simulink model "sim_MPC_Heli"  (R2020a)
settings: Solver=ode4  StartTime=0.0  StopTime=inf  FixedStep=0.01  RelTol=1e-3
InitFcn:
  | run('initialize_system.m')
values from neighbouring files (symbols this model uses):
  Ac = [d_f1_dth,d_f1_dyw,d_f1_dw_th,d_f1_dw_yw ... (first row only)    [linearize_heli.m]
  Ad = ds.a    [initialize_system.m]
  Bc = [d_f1_Vmp,d_f1_Vmy ... (first row only)    [linearize_heli.m]
  Bd = ds.b    [initialize_system.m]
  Cc = [1,0,0,0;0,1,0,0]    [linearize_heli.m]
  Cd = ds.c    [initialize_system.m]
  th_op = -10*pi/180    (= -0.174532925199)    [initialize_system.m]
  Vmp_op = (Kyy*m_heli*g*cos(th_op)*l_cm) / (Kyy*Kpp - Kyp*Kpy)    [initialize_system.m]
  Vmy_op = (Kyp*Vmp_op) / (Kyy)    [initialize_system.m]
  w_th_op = 0    [initialize_system.m]
  w_yw_op = 0    [initialize_system.m]
  yw_op = pi/2    (= 1.57079632679)    [initialize_system.m]
undefined symbols (not defined in the file or in its folder): L
libraries: simulink_extras x2, realtime_pacer_lib x1
(part 1 of 2)
settings Model: Creator=engen  LastModifiedBy=eirik.engen

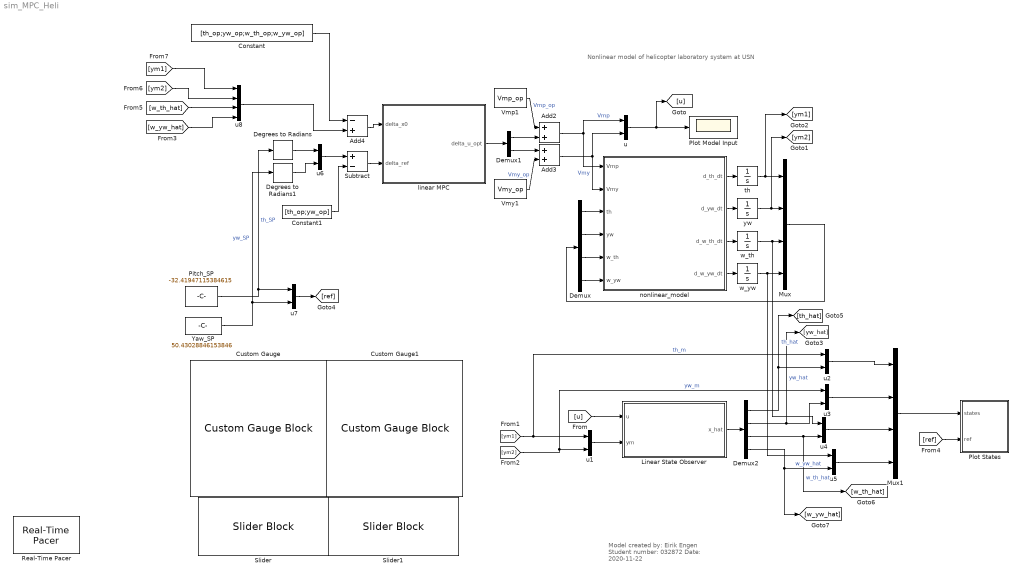
== system sim_MPC_Heli ==
  note: Model created by: Eirik Engen
      | Student number: 032872
      | Date: 2020-11-22
  note: Nonlinear model of helicopter laboratory system at USN
  Add2 : Sum
  Add3 : Sum
  Add4 : Sum  Inputs=-+
  Constant : Constant  Value=[th_op;yw_op;w_th_op;w_yw_op]
  Constant1 : Constant  Value=[th_op;yw_op]
  Custom Gauge : CustomGaugeBlock  NeedleImage=data:image/svg+xml;base64,PD94bWwgdmVyc2lvbj0iMS4wIiBlbmNvZGluZz0idXRmLTgiPz4KPCEtLSBHZW5lcmF0b3I6IEFkb2JlIElsbHVzdHJhdG9yIDE5LjIuMSwgU1ZHIEV4cG9ydCBQbHVnLUluIC4gU1ZHIFZlcnNpb246IDYuMDAgQnVpbGQgMCkgIC0tPgo8c3ZnIHZlcnNpb249IjEuMSIgeG1sbnM9Imh0dHA6Ly93d3cudzMub3JnLzIwMDAvc3ZnIiB4bWxuczp4bGluaz0iaHR0cDovL3d3dy53My5vcmcvMTk5OS94bGluayIgeD0iMHB4IiB5PSIwcHgiCgkgdmlld0JveD0iMCAwIDIwMCA1MCIgc3R5bGU9ImVuYWJsZS1iYWNrZ3JvdW5kOm5ldyAw ...(+9940 chars)  NeedleXPos=0.3917048004629798  NeedleYPos=0.48297683576593553  NeedleHeight=0.10490569201603189  NeedleWidth=0.17282438115971865  NeedleInitialRotation=-59.94322499147643  BackgroundImage=data:image/svg+xml;base64,PD94bWwgdmVyc2lvbj0iMS4wIiBlbmNvZGluZz0iVVRGLTgiIHN0YW5kYWxvbmU9Im5vIj8+CjwhLS0gR2VuZXJhdG9yOiBBZG9iZSBJbGx1c3RyYXRvciAxOS4yLjEsIFNWRyBFeHBvcnQgUGx1Zy1JbiAuIFNWRyBWZXJzaW9uOiA2LjAwIEJ1aWxkIDApICAtLT4KCjxzdmcKICAgeG1sbnM6ZGM9Imh0dHA6Ly9wdXJsLm9yZy9kYy9lbGVtZW50cy8xLjEvIgogICB4bWxuczpjYz0iaHR0cDovL2NyZWF0aXZlY29tbW9ucy5vcmcvbnMjIgogICB4bWxuczpyZGY9Imh0dHA6Ly93d3cudzMub3JnLzE5OTkvMDIvMjItcmRmLXN5bnRh ...(+9660 chars)  GaugeMax=5  GaugeArcDefined=true  GaugeArcRadius=0.12284021706659631  GaugeArcStrokeWidth=0.03592322137076783  GaugeArcRotation=240.5385250290321  GaugeArcRatio=0.8333333333333  GaugeArcTransparency=0  ValueArcColor=#1759b0  GaugeTickColor=#faf5c8  ScaleColorsJSON="[{\"Min\":0,\"Max\":1.1,\"Color\":[1,1,0]},{\"Min\":1.1,\"Max\":1.4,\"Color\":[0,1,0]},{\"Min\":1.4,\"Max\":5,\"Color\":[1,1,0]}]"  fixedAspectRatio=on  IsLinearGauge=false  GaugeTrackLeft=0.35  GaugeTrackTop=0.35  GaugeTrackHeight=0.1  GaugeTrackWidth=0.3  GaugeTrackRotation=0
  Custom Gauge1 : CustomGaugeBlock  NeedleImage=data:image/svg+xml;base64,PD94bWwgdmVyc2lvbj0iMS4wIiBlbmNvZGluZz0idXRmLTgiPz4KPCEtLSBHZW5lcmF0b3I6IEFkb2JlIElsbHVzdHJhdG9yIDE5LjIuMSwgU1ZHIEV4cG9ydCBQbHVnLUluIC4gU1ZHIFZlcnNpb246IDYuMDAgQnVpbGQgMCkgIC0tPgo8c3ZnIHZlcnNpb249IjEuMSIgeG1sbnM9Imh0dHA6Ly93d3cudzMub3JnLzIwMDAvc3ZnIiB4bWxuczp4bGluaz0iaHR0cDovL3d3dy53My5vcmcvMTk5OS94bGluayIgeD0iMHB4IiB5PSIwcHgiCgkgdmlld0JveD0iMCAwIDIwMCA1MCIgc3R5bGU9ImVuYWJsZS1iYWNrZ3JvdW5kOm5ldyAw ...(+9940 chars)  NeedleXPos=0.3917048004629798  NeedleYPos=0.48297683576593553  NeedleHeight=0.10490569201603189  NeedleWidth=0.17282438115971865  NeedleInitialRotation=-59.94322499147643  BackgroundImage=data:image/svg+xml;base64,PD94bWwgdmVyc2lvbj0iMS4wIiBlbmNvZGluZz0iVVRGLTgiIHN0YW5kYWxvbmU9Im5vIj8+CjwhLS0gR2VuZXJhdG9yOiBBZG9iZSBJbGx1c3RyYXRvciAxOS4yLjEsIFNWRyBFeHBvcnQgUGx1Zy1JbiAuIFNWRyBWZXJzaW9uOiA2LjAwIEJ1aWxkIDApICAtLT4KCjxzdmcKICAgeG1sbnM6ZGM9Imh0dHA6Ly9wdXJsLm9yZy9kYy9lbGVtZW50cy8xLjEvIgogICB4bWxuczpjYz0iaHR0cDovL2NyZWF0aXZlY29tbW9ucy5vcmcvbnMjIgogICB4bWxuczpyZGY9Imh0dHA6Ly93d3cudzMub3JnLzE5OTkvMDIvMjItcmRmLXN5bnRh ...(+9660 chars)  GaugeMax=5  GaugeArcDefined=true  GaugeArcRadius=0.12284021706659631  GaugeArcStrokeWidth=0.03592322137076783  GaugeArcRotation=240.5385250290321  GaugeArcRatio=0.8333333333333  GaugeArcTransparency=0  ValueArcColor=#1759b0  GaugeTickColor=#faf5c8  ScaleColorsJSON="[{\"Min\":0,\"Max\":0.4,\"Color\":[1,1,0]},{\"Min\":0.4,\"Max\":1.3,\"Color\":[0,1,0]},{\"Min\":1.3,\"Max\":5,\"Color\":[1,1,0]}]"  fixedAspectRatio=on  IsLinearGauge=false  GaugeTrackLeft=0.35  GaugeTrackTop=0.35  GaugeTrackHeight=0.1  GaugeTrackWidth=0.3  GaugeTrackRotation=0
  Degrees to Radians : simulink_extras/Transformations/Degrees to Radians
  Degrees to Radians1 : simulink_extras/Transformations/Degrees to Radians
  Demux : Demux
  Demux1 : Demux  Outputs=2
  Demux2 : Demux
  Linear State Observer : Subsystem
  Mux : Mux
  Mux1 : Mux
  Pitch_SP : Constant  Value=-32.41947115384615  SampleTime=-1
  Plot Model Input : Scope
  Plot States : Subsystem
  Real-Time Pacer : realtime_pacer_lib/Real-Time Pacer  simTimePerRealTime=1
  Slider : SliderBlock  ScaleMin=-45  ScaleMax=45  TickInterval=15
  Slider1 : SliderBlock  ScaleMax=180  TickInterval=20
  Subtract : Sum  Inputs=+-
  Vmp1 : Constant  Value=Vmp_op  SampleTime=-1
  Vmy1 : Constant  Value=Vmy_op  SampleTime=-1
  Yaw_SP : Constant  Value=50.43028846153846  SampleTime=-1
  linear MPC : Subsystem
  nonlinear_model : MATLAB Function  TreatAsAtomicUnit=on
  th : Integrator  InitialCondition=-10*pi/180  LimitOutput=on  UpperSaturationLimit=45*pi/180  LowerSaturationLimit=-45*pi/180  ContinuousStateAttributes='th'
  u{,1..7} (8 alike) : Mux  Inputs=2
  u8 : Mux
  w_th : Integrator  ContinuousStateAttributes='w_th'
  w_yw : Integrator  ContinuousStateAttributes='w_yw'
  yw : Integrator  InitialCondition=pi/2  LimitOutput=on  UpperSaturationLimit=180*pi/180  LowerSaturationLimit=0  ContinuousStateAttributes='yw'
  wires:
  nonlinear_model/1(d_th_dt) -> th/1
  nonlinear_model/2(d_yw_dt) -> yw/1
  nonlinear_model/3(d_w_th_dt) -> w_th/1
  nonlinear_model/4(d_w_yw_dt) -> w_yw/1
  th/1 -> [ym1], Mux/1
  yw/1 -> [ym2], Mux/2
  w_th/1 -> u4/1, Mux/3
  w_yw/1 -> u5/1, Mux/4
  Mux/1 -> Demux/1
  Demux/1 -> nonlinear_model/3(th)
  Demux/2 -> nonlinear_model/4(yw)
  Demux/3 -> nonlinear_model/5(w_th)
  Demux/4 -> nonlinear_model/6(w_yw)
  u/1 -> [u], Plot Model Input/1
  [u] -> Linear State Observer/1(u)
  u1/1 -> Linear State Observer/2(ym)
  Linear State Observer/1(x_hat) -> Demux2/1
  Mux1/1 -> Plot States/1(states)
  u2/1 -> Mux1/1
  u3/1 -> Mux1/2
  Demux2/1 -> [th_hat], u2/2  "th_hat"
  Demux2/2 -> [yw_hat], u3/2  "yw_hat"
  u5/1 -> Mux1/4
  u4/1 -> Mux1/3
  [ym1] -> u2/1, u1/1  "th_m"
  Demux2/4 -> [w_yw_hat], u5/2  "w_yw_hat"
  Demux2/3 -> [w_th_hat], u4/2  "w_th_hat"
  [ym2] -> u3/1, u1/2  "yw_m"
  linear MPC/1(delta_u_opt) -> Demux1/1
  Demux1/2 -> Add3/1
  Demux1/1 -> Add2/2
  Vmy1/1 -> Add3/2  "Vmy_op"
  Vmp1/1 -> Add2/1  "Vmp_op"
  Add2/1 -> nonlinear_model/1(Vmp), u/1  "Vmp"
  Add3/1 -> nonlinear_model/2(Vmy), u/2  "Vmy"
  Constant/1 -> Add4/1
  Add4/1 -> linear MPC/1(delta_x0)
  Constant1/1 -> Subtract/2
  Subtract/1 -> linear MPC/2(delta_ref)
  u6/1 -> Subtract/1
  Pitch_SP/1 -> Degrees to Radians/1, u7/1  "th_SP"
  Yaw_SP/1 -> u7/2, Degrees to Radians1/1  "yw_SP"
  Degrees to Radians/1 -> u6/1
  Degrees to Radians1/1 -> u6/2
  u7/1 -> [ref]
  [ref] -> Plot States/2(ref)
  u8/1 -> Add4/2
  [ym1] -> u8/1
  [ym2] -> u8/2
  [w_th_hat] -> u8/3
  [w_yw_hat] -> u8/4

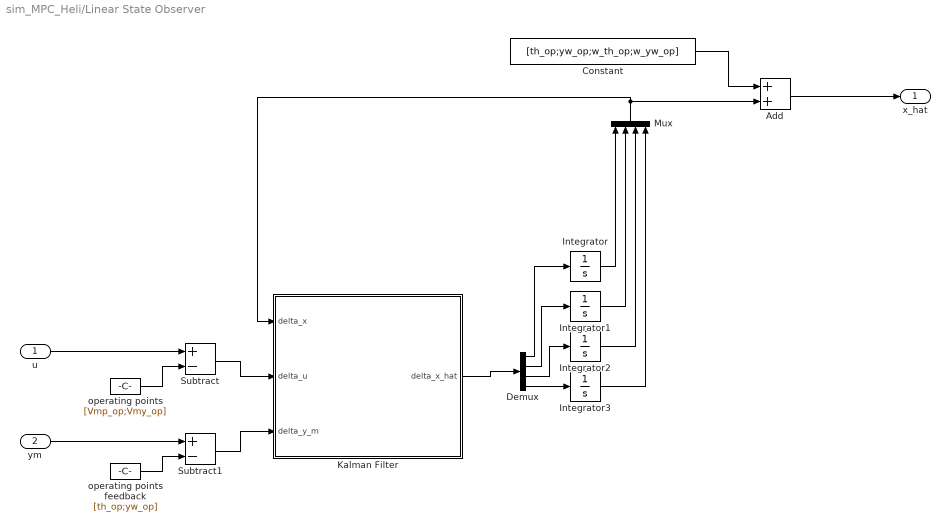
== system sim_MPC_Heli/Linear State Observer ==
  u : Inport
  ym : Inport  Port=2
  Add : Sum
  Constant : Constant  Value=[th_op;yw_op;w_th_op;w_yw_op]
  Demux : Demux
  Integrator{,1..3} (4 alike) : Integrator
  Kalman Filter : MATLAB Function  TreatAsAtomicUnit=on
  Mux : Mux
  Subtract : Sum  Inputs=+-
  Subtract1 : Sum  Inputs=+-
  operating points : Constant  Value=[Vmp_op;Vmy_op]
  operating points feedback : Constant  Value=[th_op;yw_op]
  x_hat : Outport
  wires:
  Kalman Filter/1(delta_x_hat) -> Demux/1
  u/1 -> Subtract/1
  operating points/1 -> Subtract/2
  Subtract/1 -> Kalman Filter/2(delta_u)
  Mux/1 -> Kalman Filter/1(delta_x), Add/2
  Demux/1 -> Integrator/1
  Demux/2 -> Integrator1/1
  Demux/3 -> Integrator2/1
  Demux/4 -> Integrator3/1
  Integrator/1 -> Mux/1
  Integrator1/1 -> Mux/2
  Integrator2/1 -> Mux/3
  Integrator3/1 -> Mux/4
  Subtract1/1 -> Kalman Filter/3(delta_y_m)
  ym/1 -> Subtract1/1
  operating points feedback/1 -> Subtract1/2
  Constant/1 -> Add/1
  Add/1 -> x_hat/1

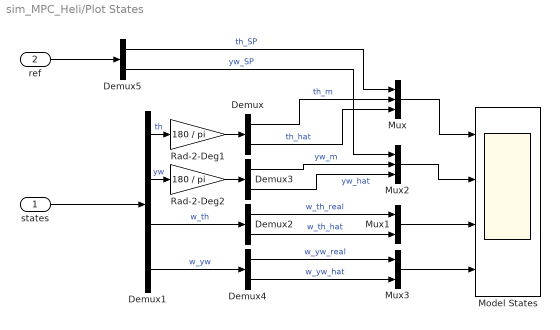
== system sim_MPC_Heli/Plot States ==
  states : Inport
  ref : Inport  Port=2
  Demux{,2..5} (5 alike) : Demux  Outputs=2
  Demux1 : Demux
  Model States : Scope  NumInputPorts=4
  Mux : Mux  Inputs=3
  Mux1 : Mux  Inputs=2
  Mux2 : Mux  Inputs=3
  Mux3 : Mux  Inputs=2
  Rad-2-Deg1 : Gain  Gain=180 / pi
  Rad-2-Deg2 : Gain  Gain=180 / pi
  wires:
  states/1 -> Demux1/1
  Demux/1 -> Mux/2  "th_m"
  Demux/2 -> Mux/3  "th_hat"
  Demux3/1 -> Mux2/2  "yw_m"
  Demux3/2 -> Mux2/3  "yw_hat"
  Demux2/1 -> Mux1/1  "w_th_real"
  Demux2/2 -> Mux1/2  "w_th_hat"
  Demux4/1 -> Mux3/1  "w_yw_real"
  Demux4/2 -> Mux3/2  "w_yw_hat"
  Demux1/1 -> Rad-2-Deg1/1  "th"
  Demux1/2 -> Rad-2-Deg2/1  "yw"
  Demux1/3 -> Demux2/1  "w_th"
  Demux1/4 -> Demux4/1  "w_yw"
  Mux/1 -> Model States/1
  Mux2/1 -> Model States/2
  Mux1/1 -> Model States/3
  Mux3/1 -> Model States/4
  ref/1 -> Demux5/1
  Demux5/2 -> Mux2/1  "yw_SP"
  Demux5/1 -> Mux/1  "th_SP"
  Rad-2-Deg1/1 -> Demux/1
  Rad-2-Deg2/1 -> Demux3/1
